simulink model "KukaSimModel_SO"  (R2021a)
settings: Solver=VariableStepAuto  StartTime=0.0  StopTime=36  FixedStep=0.01  RelTol=1e-3
PreLoadFcn:
  | TP_TASK_SPACE = Simulink.Variant('TP_MODE==1');
  | TP_JOINT_SPACE = Simulink.Variant('TP_MODE==2');
InitFcn:
  | if TP_MODE == 1
  |     %pass
  |     return;
  | end
  | jointWaypoints = zeros(4, size(waypoints, 2));
  | for i=1:size(waypoints, 2)
  |     config = FBR.searchConfiguration( ...
  |         FBR.solveIK(bodyLengths.La, bodyLengths.Lb, bodyLengths.Lc, waypoints(1, i), waypoints(2, i)) ...
  |     );
  |     jointWaypoints(:, i) = [config.th1; config.th2; config.th3; config.th4];
  | end
undefined symbols (not defined in the file): dhParametersStruct, dt_FixedStep, dynamicAttr, dynamicProps, q1, q2, q3, q4, q5, q6, waypoints, waypointTimes
libraries: robotcorelib x2
settings Model: Creator=chiar  LastModifiedBy=chiar
settings OptimizationCC: BlockReduction=off  DefaultParameterBehavior=Inlined  BufferReuse=off
settings GRTTargetCC: RTWCAPISignals=on  RTWCAPIParams=on

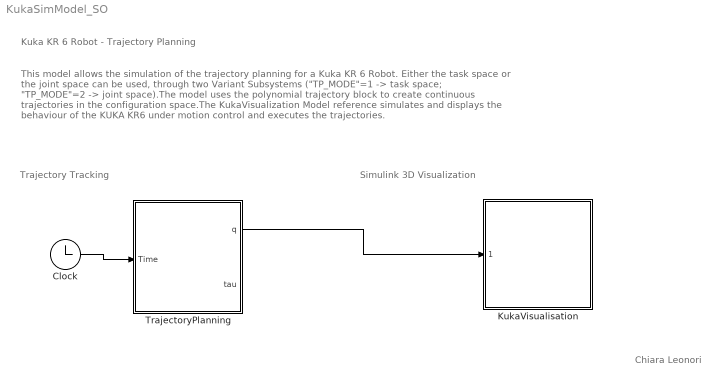
== system KukaSimModel_SO ==
  note: Chiara Leonori
  note: Trajectory Tracking
  note: Simulink 3D Visualization
  note: This model allows the simulation of the trajectory planning for a Kuka KR 6 Robot. Either the task space or the joint space can be used, through two Variant Subsystems ("TP_MODE"=1 -> task space; "TP_MODE"=2 -> joint space).The model uses the polynomial trajectory block to create continuous trajectories in the configuration space.The KukaVisualization Model reference simulates and displays the behaviour of the KUKA KR6 under motion control and executes the trajectories.
  note: Kuka KR 6 Robot - Trajectory Planning
  Clock : Clock
  KukaVisualisation : Subsystem  ReferencedSubsystem=KukaVisualisationModel
  TrajectoryPlanning : Subsystem  Variant=on
  wires:
  TrajectoryPlanning/1(q) -> KukaVisualisation/1
  Clock/1 -> TrajectoryPlanning/1(Time)

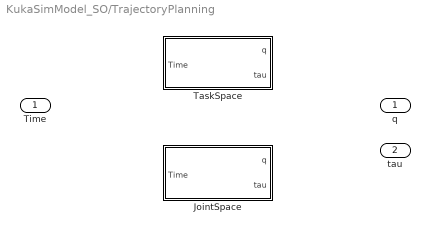
== system KukaSimModel_SO/TrajectoryPlanning ==
  Time : Inport
  JointSpace : Subsystem  VariantControl=TP_MODE == 2
  TaskSpace : Subsystem  VariantControl=TP_MODE == 1
  q : Outport  OutDataTypeStr=Bus: Bus_q
  tau : Outport  Port=2  OutDataTypeStr=double

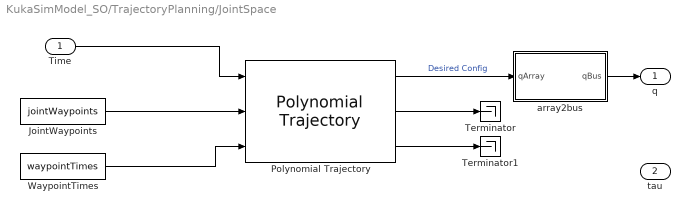
== system KukaSimModel_SO/TrajectoryPlanning/JointSpace ==
  Time : Inport
  JointWaypoints : Constant  Value=jointWaypoints
  Polynomial Trajectory : robotcorelib/Polynomial Trajectory  WaypointSource=External  Waypoints=[ 0, 2, 1, 5, 0; -1, 3, 1, 4, 4 ]  TimePoints=[ 0, 1, 2, 3, 4 ]  TimeInterval=[ 1, 4 ]  Method=Cubic Polynomial  ParameterSource=Internal  VelocityBoundaryCondition=zeros( 4, size(waypoints, 2) )  AccelerationBoundaryCondition=zeros( 2, 5 )  SimulateUsing=Interpreted execution
  Terminator : Terminator
  Terminator1 : Terminator
  WaypointTimes : Constant  Value=waypointTimes
  array2bus : MATLAB Function  TreatAsAtomicUnit=on
  q : Outport  OutDataTypeStr=Bus: Bus_q
  tau : Outport  Port=2  OutDataTypeStr=double
  wires:
  Time/1 -> Polynomial Trajectory/1
  Polynomial Trajectory/2 -> Terminator/1
  Polynomial Trajectory/3 -> Terminator1/1
  WaypointTimes/1 -> Polynomial Trajectory/3
  Polynomial Trajectory/1 -> array2bus/1(qArray)  "Desired Config"
  array2bus/1(qBus) -> q/1
  JointWaypoints/1 -> Polynomial Trajectory/2

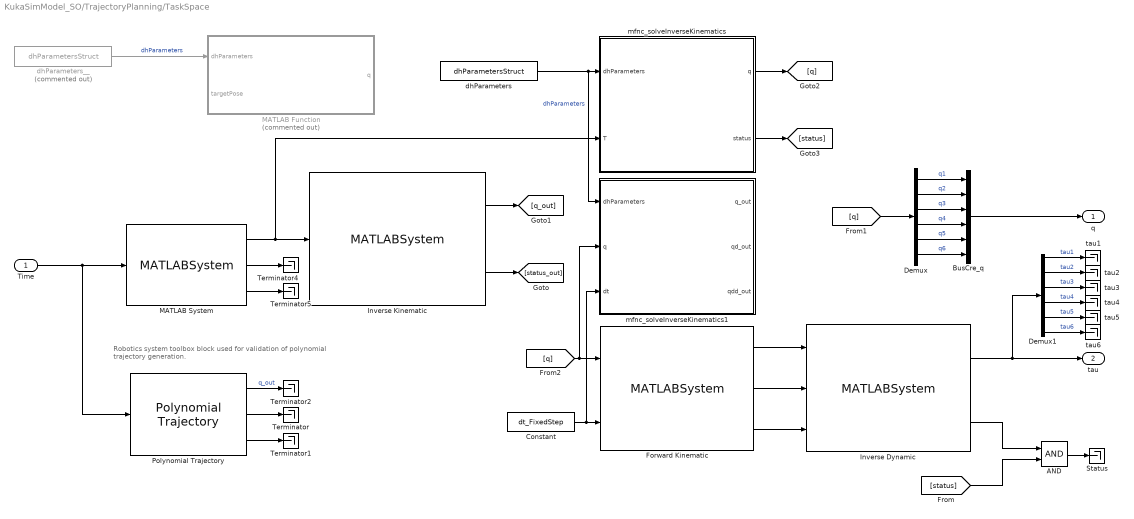
== system KukaSimModel_SO/TrajectoryPlanning/TaskSpace ==
  note: Robotics system toolbox block used for validation
      | of polynomial trajectory generation.
  Time : Inport
  AND : Logic  AllPortsSameDT=off  OutDataTypeStr=boolean
  BusCre_q : BusCreator  Inputs=q1,q2,q3,q4,q5,q6  OutDataTypeStr=Bus: Bus_q
  Constant : Constant  Value=dt_FixedStep  OutDataTypeStr=double
  Demux : Demux  Outputs=6
  Demux1 : Demux  Outputs=6
  Forward Kinematic : MATLABSystem  System=core.Kuka6  Solver=Forward Kinematic  DHStruct=dhParametersStruct  Tolerance=1e-6  M=dynamicProps.M  I=dynamicProps.I  Fext=zeros( 6, 1 )  SimulateUsing=Interpreted execution
      mask Type: core.Kuka6
      mask Display:
      | image('srcs\simulink\blockicons\solver-fk-icon.jpg');
      | port_label('input',1,'q');
      | port_label('input',2,'dt');
      | port_label('output',1,'q_out');
      | port_label('output',2,'qd_out');
      | port_label('output',3,'qdd_out');
  Inverse Dynamic : MATLABSystem  System=core.Kuka6  Solver=Inverse Dynamic  DHStruct=dhParametersStruct  Tolerance=1e-6  M=dynamicAttr.M  I=dynamicAttr.I  Fext=zeros( 6, 1 )  SimulateUsing=Interpreted execution
      mask Type: core.Kuka6
      mask Display:
      | image('srcs\simulink\blockicons\solver-id-icon.jpg');
      | port_label('input',1,'q');
      | port_label('input',2,'qd');
      | port_label('input',3,'qdd');
      | port_label('output',1,'tau');
      | port_label('output',2,'status');
  Inverse Kinematic : MATLABSystem  System=core.Kuka6  Solver=Inverse Kinematic  DHStruct=dhParametersStruct  Tolerance=1e-6  M=zeros( 6, 1 )  I=zeros( 3, 3, 6 )  Fext=zeros( 6, 1 )  SimulateUsing=Interpreted execution
      mask Type: core.Kuka6
      mask Display:
      | image('srcs\simulink\blockicons\solver-ik-icon.jpg');
      | port_label('input',1,'targetPose');
      | port_label('output',1,'q');
      | port_label('output',2,'status');
  MATLAB Function : MATLAB Function  Commented=on  TreatAsAtomicUnit=on
  MATLAB System : MATLABSystem  System=core.TrajectoryGenerator  Method=Quintic Polynomial  Waypoints=waypointsStruct.waypoints  Timepoints=waypointsStruct.times  Velocities=waypointsStruct.velocities  Accelerations=waypointsStruct.accelerations  SimulateUsing=Interpreted execution
      mask Type: core.TrajectoryGenerator
      mask Display:
      | image('srcs\simulink\blockicons\polynomial-icon-big.jpg');
      | port_label('input',1,'t');
      | port_label('output',1,'q_out');
      | port_label('output',2,'qd_out');
      | port_label('output',3,'qdd_out');
  Polynomial Trajectory : robotcorelib/Polynomial Trajectory  WaypointSource=Internal  Waypoints=waypoints  TimePoints=waypointTimes  TimeInterval=[ 1, 4 ]  Method=Quintic Polynomial  ParameterSource=Internal  VelocityBoundaryCondition=waypointVels  AccelerationBoundaryCondition=waypointAccels  SimulateUsing=Interpreted execution
  Status : Terminator
  Terminator{,1..2,4..5} (5 alike) : Terminator
  dhParameters : Constant  Value=dhParametersStruct  OutDataTypeStr=Bus: Bus_dhParameter
  dhParameters__ : Constant  Commented=on  Value=dhParametersStruct  OutDataTypeStr=Bus: Bus_dhParameter
  mfnc_solveInverseKinematics : MATLAB Function  TreatAsAtomicUnit=on
  mfnc_solveInverseKinematics1 : MATLAB Function  TreatAsAtomicUnit=on
  tau{1..6} (6 alike) : Terminator
  q : Outport  OutDataTypeStr=Bus: Bus_q
  tau : Outport  Port=2  OutDataTypeStr=double
  wires:
  Time/1 -> Polynomial Trajectory/1, MATLAB System/1
  Polynomial Trajectory/2 -> Terminator/1
  Polynomial Trajectory/3 -> Terminator1/1
  Polynomial Trajectory/1 -> Terminator2/1  "q_out"
  dhParameters__/1 -> MATLAB Function/1(dhParameters)  "dhParameters"
  Inverse Dynamic/1 -> Demux1/1, tau/1
  MATLAB System/2 -> Terminator4/1
  MATLAB System/3 -> Terminator5/1
  Demux/1 -> BusCre_q/1  "q1"
  Demux/2 -> BusCre_q/2  "q2"
  Demux/3 -> BusCre_q/3  "q3"
  Demux/4 -> BusCre_q/4  "q4"
  Demux/5 -> BusCre_q/5  "q5"
  Demux/6 -> BusCre_q/6  "q6"
  BusCre_q/1 -> q/1
  MATLAB System/1 -> mfnc_solveInverseKinematics/2(T), Inverse Kinematic/1
  Forward Kinematic/1 -> Inverse Dynamic/1
  Forward Kinematic/2 -> Inverse Dynamic/2
  Forward Kinematic/3 -> Inverse Dynamic/3
  Inverse Dynamic/2 -> AND/1
  AND/1 -> Status/1
  Constant/1 -> mfnc_solveInverseKinematics1/3(dt), Forward Kinematic/2
  Inverse Kinematic/2 -> [status_out]
  [status] -> AND/2
  Inverse Kinematic/1 -> [q_out]
  [q] -> Demux/1
  [q] -> mfnc_solveInverseKinematics1/2(q), Forward Kinematic/1
  Demux1/1 -> tau1/1  "tau1"
  Demux1/2 -> tau2/1  "tau2"
  Demux1/3 -> tau3/1  "tau3"
  Demux1/4 -> tau4/1  "tau4"
  Demux1/5 -> tau5/1  "tau5"
  Demux1/6 -> tau6/1  "tau6"
  dhParameters/1 -> mfnc_solveInverseKinematics1/1(dhParameters), mfnc_solveInverseKinematics/1(dhParameters)  "dhParameters"
  mfnc_solveInverseKinematics/1(q) -> [q]
  mfnc_solveInverseKinematics/2(status) -> [status]

== matlab function KukaSimModel_SO/TrajectoryPlanning/TaskSpace/mfnc_solveInverseKinematics ==
  data: dhParameters input; T input; q output; status output
function [q, status] = solveInverseKinematics(dhParameters, T)
% initialize output
q = zeros(6, 1); status = cast(0, 'int8');

dim = size(T);
if (dim(1) == 3 && dim(2) == 1) || ...
        (dim(1) == 1 && dim(2) == 3)
    % define homogeneous transform T from pose
    TT = [1, 0, 0, T(1, 1);
        0, -1, 0, T(2, 1);
        0, 0, -1, T(3, 1);
        0, 0, 0, 1];
else 
    TT = T;
end
[q, status] = solver.solveInverseKinematics(dhParameters, TT);
end

== matlab function KukaSimModel_SO/TrajectoryPlanning/TaskSpace/MATLAB Function ==
  data: dhParameters input Bus: Bus_dhParameter; targetPose input double size=[3 1]; q output Bus: Bus_q
function q = IKSolver(dhParameters, targetPose)
T = [1, 0, 0, targetPose(1, 1);
    0, -1, 0, targetPose(2, 1);
    0, 0, -1, targetPose(3, 1);
    0, 0, 0, 1];
sixAxesRobot = SixAxesRobot(dhParameters);
sixAxesRobot.disableVerbose();
solution = sixAxesRobot.solveIK(T);

q.q1 = solution(1);
q.q2 = solution(2);
q.q3 = solution(3);
q.q4 = solution(4);
q.q5 = solution(5);
q.q6 = solution(6);

== matlab function KukaSimModel_SO/TrajectoryPlanning/JointSpace/array2bus ==
  data: qArray input; qBus output Bus: Bus_q
function qBus = adapter(qArray)
    qBus.th1 = qArray(1);
    qBus.th2 = qArray(2);
    qBus.th3 = qArray(3);
    qBus.th4 = qArray(4);

== matlab function KukaSimModel_SO/TrajectoryPlanning/TaskSpace/mfnc_solveInverseKinematics1 ==
  data: dhParameters input; q input; q_out output; qd_out output; dt input; qdd_out output
function [q_out, qd_out, qdd_out] = solveForwardKinematics(dhParameters, q, dt)
coder.internal.errorIf(nargin > 2 & nargout < 3, 'solver:solveForwardKinematics:NotEnoughInputArgument');
n = 6;
y = zeros(3, n);
T = eye(4, 4); % initialize T for first computation
for i=1:n
    T = T*solver.computeT(dhParameters(i, :), q(i));
    y(:, i) = T(1:3, 4);
end
if nargout > 1 && nargin > 2 % if dt is given and gradient can be calculated
    q_out = y;
    qd_out = gradient(q_out, dt);
    qdd_out = gradient(qd_out, dt);
else
    q_out = T;
    qd_out = zeros(3, n);
    qdd_out = zeros(3, n);
end
end
